simulink model "bt3"  (R2019a)
settings: Solver=ode4  StartTime=0.0  StopTime=1500  FixedStep=0.1  RelTol=1e-3
model workspace (MAT data in the model file):
  k0 = Simulink.Parameter
  k0.DataType = 'auto'
  k0.Dimensions = [0 0]
undefined symbols (not defined in the file): sigbuilder_block
libraries: fuzblock x1
settings Model: Creator=ASUS  LastModifiedBy=ASUS

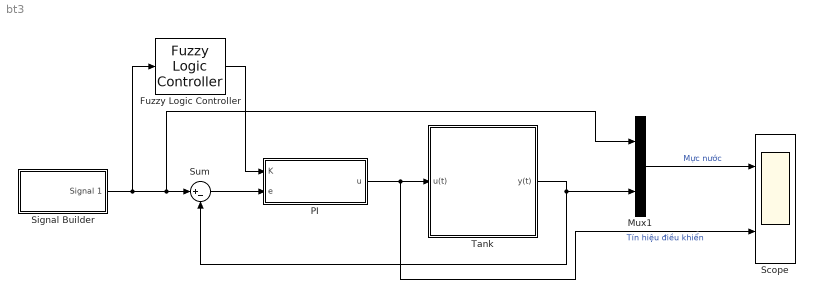
== system bt3 ==
  Fuzzy Logic Controller : fuzblock/Fuzzy Logic  Controller  FIS='FuzzySugenoPID_SingleTank.fis'  OutputSampleNumber=101  DataType=double  FuzzifiedInputs=off  RuleFiringStrengths=off  RuleOutputs=off  AggregatedOutputs=off  SimulateUsing=Interpreted execution  OutOfRangeInputValueMessage=warning  NoRuleFiredMessage=warning  EmptyOutputFuzzySetMessage=warning
  Mux1 : Mux  Inputs=2
  PI : Subsystem
  Scope : Scope  NumInputPorts=2
  Signal Builder : Subsystem  Tag=STV Subsys  LoadFcn=sigbuilder_block('load');  StartFcn=sigbuilder_block('start');  StopFcn=sigbuilder_block('stop');  ClipboardFcn=sigbuilder_block('clipboard');  mask(Sigbuilder block){tuvar=[0:10]}
      mask help: Simulink:masks:SigbuilderBlock_MD
      mask init:
      | if ~strcmp(get_param(bdroot(gcbh),'SimulationStatus'),'stopped') tuvar = sigbuilder_block('maskInit'); end
      settings: CopyFcn=sigbuilder_block('copy');  DeleteFcn=sigbuilder_block('delete');  ModelCloseFcn=sigbuilder_block('modelClose');  PreSaveFcn=sigbuilder_block('preSave');  PauseFcn=sigbuilder_block('pause');  ContinueFcn=sigbuilder_block('continue');  NameChangeFcn=sigbuilder_block('namechange');  OpenFcn=sigbuilder_block('open',[437.6 199.2 550.4 400 ]);  CloseFcn=sigbuilder_block('close');
      mask Display: plot(0, 0, 100, 100,[2, 2, 32, 32, 2], [68, 8, 8, 68, 68],[32, 2], [38, 38], [32, 19, 2],[53, 60, 44], [32, 17, 17, 2],[16, 16, 31, 31]);txt = getActiveGroup(gcbh);text(2, 100, txt,'verticalAlignment', 'top');
  Sum : Sum  Inputs=|+-
  Tank : Subsystem  mask{r_max=20, r_min=10, y_max=100, y_min=0, K=50, b=1.5, C=0.8, g=981}
      mask prompts: r_max "r max"; r_min "r min"; y_max "y max"; y_min "y min"
      mask Display: image(imread('bt3.png'))
  wires:
  Signal Builder/1(Signal 1) -> Fuzzy Logic Controller/1, Mux1/1, Sum/1
  Mux1/1 -> Scope/1  "Mực nước"
  Tank/1(y(t)) -> Mux1/2, Sum/2
  PI/1(u) -> Scope/2, Tank/1(u(t))  "Tín hiệu điều khiển"
  Sum/1 -> PI/2(e)
  Fuzzy Logic Controller/1 -> PI/1(K)

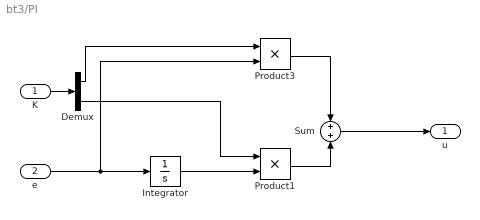
== system bt3/PI ==
  K : Inport
  e : Inport  Port=2
  Demux : Demux  Outputs=2
  Integrator : Integrator
  Product1 : Product
  Product3 : Product
  Sum : Sum
  u : Outport
  wires:
  K/1 -> Demux/1
  e/1 -> Product3/2, Integrator/1
  Demux/2 -> Product1/1
  Integrator/1 -> Product1/2
  Product3/1 -> Sum/1
  Demux/1 -> Product3/1
  Product1/1 -> Sum/2
  Sum/1 -> u/1

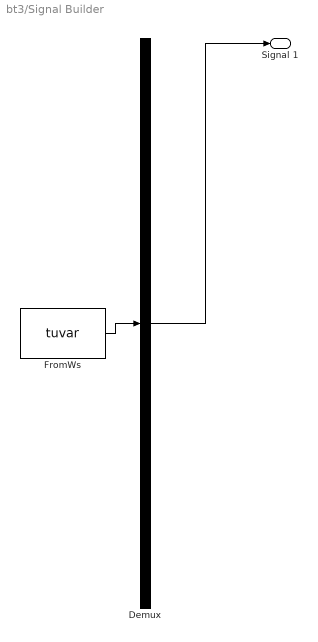
== system bt3/Signal Builder ==
  Demux : Demux  Tag=STV Demux  Outputs=1
  FromWs : FromWorkspace  Tag=STV FromWs  VariableName=tuvar  SampleTime=0
      SigBuilderData=|
      | common.afterFinalStr = 'Extrapolate'
      | common.sampleTime = 0
      | dataSet.timeRange = [0 1500]
      | dataSet.name = 'Group 1'
      | sbobj.Groups.Name = 'Group 1'
      | sbobj.Groups.Signals.Name = 'Signal 1'
      | sbobj.Groups.Signals.XData = [0 180 180 465 465 725 725 985 985 1250 1250 1500]
      | sbobj.Groups.Signals.YData = [100 100 0 0 26.5 26.5 49.5 49.5 30 30 90 90]
      | sbobj.Groups.TimeRange = [0 1500]
  Signal 1 : Outport  Tag=STV Outport
  wires:
  Demux/1 -> Signal 1/1
  FromWs/1 -> Demux/1

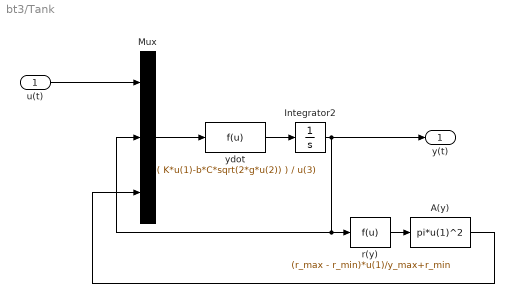
== system bt3/Tank ==
  u(t) : Inport
  A(y) : Fcn  Expr=pi*u(1)^2
  Integrator2 : Integrator
  Mux : Mux  Inputs=3
  r(y) : Fcn  Expr=(r_max - r_min)*u(1)/y_max+r_min
  ydot : Fcn  Expr=( K*u(1)-b*C*sqrt(2*g*u(2)) ) / u(3)
  y(t) : Outport
  wires:
  ydot/1 -> Integrator2/1
  Mux/1 -> ydot/1
  u(t)/1 -> Mux/1
  Integrator2/1 -> Mux/2, r(y)/1, y(t)/1
  A(y)/1 -> Mux/3
  r(y)/1 -> A(y)/1
